simulink model "zbiornik3"  (R2015a)
settings: Solver=ode3  StartTime=0.0  StopTime=50  FixedStep=0.01  RelTol=1e-3
values from neighbouring files (symbols this model uses):
  a3 = x2(2)    [ident1.m]
  C3 = x2(1)    [ident1.m]
  h30 = max(y3)    [ucinanie.m]
  R = 36.4    [ident1.m]    (also in wyniki_akt.mat; zbiornik_1.m; zbiornik_2.m; zbiornik_3.m)
  w = 5    [ident1.m]    (also in wyniki_akt.mat; zbiornik_1.m; zbiornik_2.m; zbiornik_3.m)
settings Model: Creator=Ziger  LastModifiedBy=Student

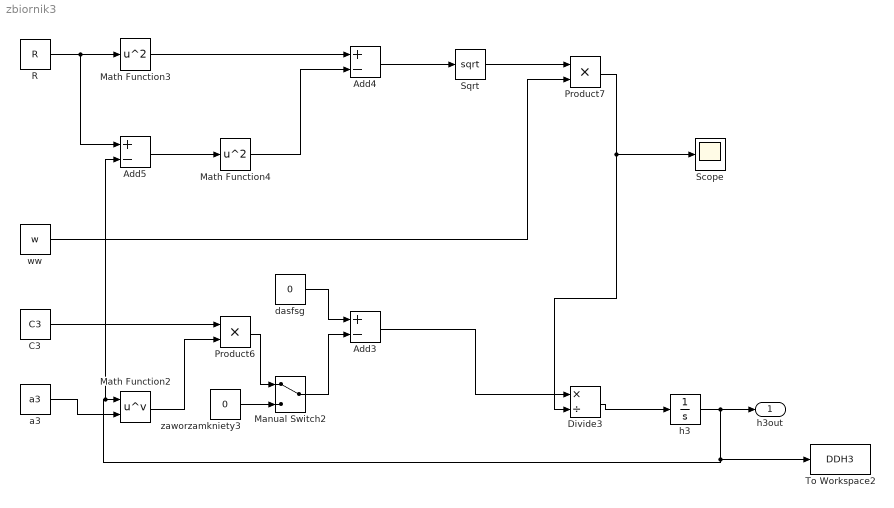
== system zbiornik3 ==
  Add3 : Sum  Inputs=+-
  Add4 : Sum  Inputs=+-
  Add5 : Sum  Inputs=+-
  C3 : Constant  Value=C3
  Divide3 : Product  Inputs=*/
  Manual Switch2 : ManualSwitch
  Math Function2 : Math  Operator=pow  SaturateOnIntegerOverflow=on
  Math Function3 : Math  Operator=square  SaturateOnIntegerOverflow=on
  Math Function4 : Math  Operator=square  SaturateOnIntegerOverflow=on
  Product6 : Product
  Product7 : Product
  R : Constant  Value=R
  Scope : Scope
  Sqrt : Sqrt  SaturateOnIntegerOverflow=on
  To Workspace2 : ToWorkspace  VariableName=DDH3  SaveFormat=Structure With Time  SampleTime=-1
  a3 : Constant  Value=a3
  dasfsg : Constant  Value=0
  h3 : Integrator  InitialCondition=h30  LimitOutput=on  UpperSaturationLimit=35  LowerSaturationLimit=0
  ww : Constant  Value=w
  zaworzamkniety3 : Constant  Value=0
  "h3out " : Outport
  wires:
  Product7/1 -> Divide3/2, Scope/1
  Add3/1 -> Divide3/1
  R/1 -> Add5/1, Math Function3/1
  h3/1 -> "h3out "/1, To Workspace2/1, Add5/2, Math Function2/1
  Math Function3/1 -> Add4/1
  Add4/1 -> Sqrt/1
  Divide3/1 -> h3/1
  Sqrt/1 -> Product7/1
  Math Function2/1 -> Product6/2
  Add5/1 -> Math Function4/1
  a3/1 -> Math Function2/2
  C3/1 -> Product6/1
  ww/1 -> Product7/2
  Math Function4/1 -> Add4/2
  Product6/1 -> Manual Switch2/1
  zaworzamkniety3/1 -> Manual Switch2/2
  Manual Switch2/1 -> Add3/2
  dasfsg/1 -> Add3/1
